simulink model "test07"  (Simulink 7.4)
settings: Solver=ode3  StartTime=0.0  StopTime=inf  RelTol=1e-3
undefined symbols (not defined in the file or in its folder): serial
libraries: instrumentlib x3, NAV420Lib x2, NAV420DecodeLib x1
settings Model: Creator=djulzz  LastModifiedBy=djulzz
settings DebuggingCC: SolverPrmCheckMsg=none

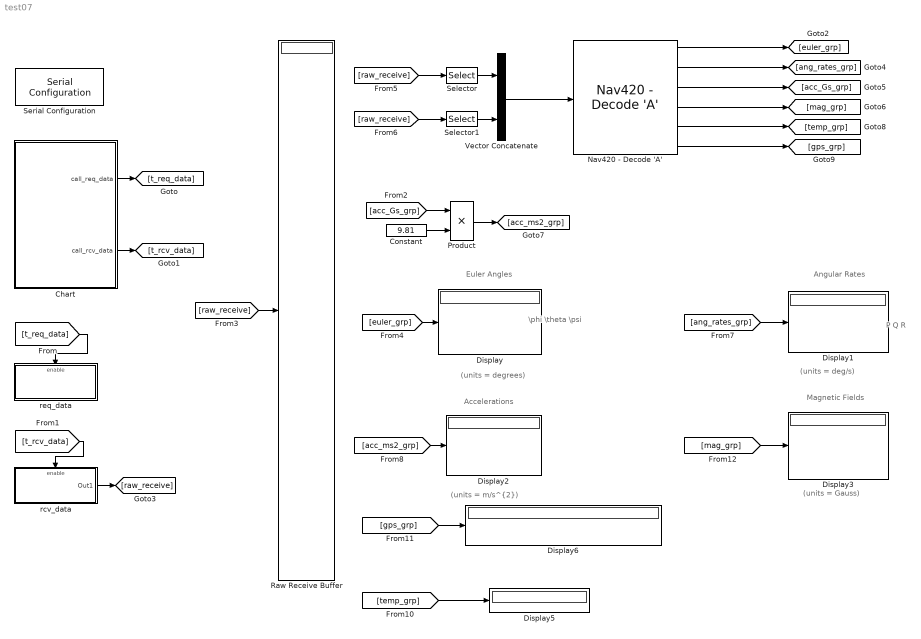
== system test07 ==
  note: \phi
      | \theta
      | \psi
  note: P
      | Q
      | R
  note: (units = degrees)
  note: Euler Angles
  note: Angular Rates
  note: (units = deg/s)
  note: Accelerations
  note: (units = m/s^{2})
  note: (units = Gauss)
  note: Magnetic Fields
  Chart : Stateflow chart
  Constant : Constant  Value=9.81  OutDataTypeMode=double  OutDataType=fixdt(1, 16)  OutScaling=2^0  OutDataTypeStr=double  SampleTime=-1
  Display{,1..3,5..6} (6 alike) : Display
  Nav420 - Decode 'A' : NAV420DecodeLib/Nav420 - Decode 'A'  SystemSampleTime=-1
  Product : Product  OutDataTypeMode=double  OutDataType=fixdt(1, 16)  OutScaling=2^0  OutDataTypeStr=double  RndMeth=Zero
  Raw Receive Buffer : Display
      settings: Format=hex (Stored Integer)  Decimation=35
  Selector : Selector  InputPortWidth=35  IndexOptions=Index vector (dialog)  Indices=[6 7 8 9 10 11 12 13 14 15 16 17 18 19 20 21 22 23 24 25 26 27 28 29 30 31 32 33 34 35]  OutputSizes=1
  Selector1 : Selector  InputPortWidth=35  IndexOptions=Index vector (dialog)  Indices=[1 2 3 4 5]  OutputSizes=1
  Serial Configuration : instrumentlib/Serial Configuration  Priority=-200000  DialogController=instrumentcreatedialog  DialogControllerArgs=DataTag0  ComPortMenu=COM1  ComPort=COM1  ObjConstructor=serial('COM1');  BaudRate=38400  DataBits=8  Parity=none  StopBits=1  FlowControl=none  Timeout=10  ByteOrder=LittleEndian
  Vector Concatenate : Concatenate  Mode=Vector
  rcv_data : Subsystem  TreatAsAtomicUnit=on
  req_data : Subsystem  TreatAsAtomicUnit=on
  wires:
  [t_req_data] -> req_data/Enable
  [t_rcv_data] -> rcv_data/Enable
  Chart/1(call_req_data) -> [t_req_data]
  Chart/2(call_rcv_data) -> [t_rcv_data]
  [raw_receive] -> Raw Receive Buffer/1
  rcv_data/1(Out1) -> [raw_receive]
  Nav420 - Decode 'A'/1 -> [euler_grp]
  [raw_receive] -> Selector/1
  [raw_receive] -> Selector1/1
  Selector1/1 -> Vector Concatenate/2
  Selector/1 -> Vector Concatenate/1
  Vector Concatenate/1 -> Nav420 - Decode 'A'/1
  Nav420 - Decode 'A'/2 -> [ang_rates_grp]
  Nav420 - Decode 'A'/3 -> [acc_Gs_grp]
  Nav420 - Decode 'A'/4 -> [mag_grp]
  Constant/1 -> Product/2
  [acc_Gs_grp] -> Product/1
  Product/1 -> [acc_ms2_grp]
  Nav420 - Decode 'A'/5 -> [temp_grp]
  Nav420 - Decode 'A'/6 -> [gps_grp]
  [euler_grp] -> Display/1
  [ang_rates_grp] -> Display1/1
  [acc_ms2_grp] -> Display2/1
  [gps_grp] -> Display6/1
  [mag_grp] -> Display3/1
  [temp_grp] -> Display5/1

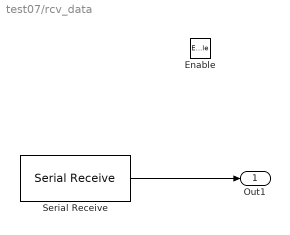
== system test07/rcv_data ==
  Enable : EnablePort
  Serial Receive : instrumentlib/Serial Receive  DialogController=instrumentcreatedialog  DialogControllerArgs=DataTag1  ComPortMenu=COM1  ComPort=COM1  ObjConstructor=serial('COM1');  Terminator=<none>  DataSize="[35   1]"  DataType=uint8  EnableBlockingMode=on  ActionDataUnavailable=Output last received value  CustomValue=0  SampleTime=-1
  Out1 : Outport  DataType=uint8  OutDataType=fixdt(1, 16)  OutScaling=2^0  OutDataTypeStr=uint8
  wires:
  Serial Receive/1 -> Out1/1

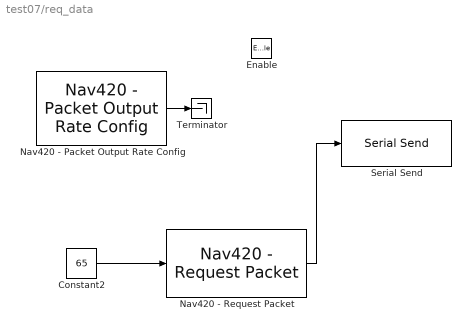
== system test07/req_data ==
  Enable : EnablePort
  Constant2 : Constant  Value=65  OutDataTypeMode=int8  OutDataType=fixdt(1, 16)  OutScaling=2^0  OutDataTypeStr=int8  SampleTime=-1
  Nav420 - Packet Output Rate Config : NAV420Lib/Nav420 - Packet Output Rate Config  SystemSampleTime=-1  shouldSave=on  output_rate=0
  Nav420 - Request Packet : NAV420Lib/Nav420 - Request Packet  SystemSampleTime=-1
  Serial Send : instrumentlib/Serial Send  DialogController=instrumentcreatedialog  DialogControllerArgs=DataTag2  ComPortMenu=COM1  ComPort=COM1  ObjConstructor=serial('COM1');  Terminator=<none>  EnableBlockingMode=on
  Terminator : Terminator
  wires:
  Constant2/1 -> Nav420 - Request Packet/1
  Nav420 - Packet Output Rate Config/1 -> Terminator/1
  Nav420 - Request Packet/1 -> Serial Send/1

== stateflow chart Chart ==
  state Step1
    call_req_data=1;
  state Step2
    call_req_data=0;
  state Step3
    call_rcv_data=1;
  state Step4
    call_rcv_data=0;
  (default) -> Step1
  Step1 -> Step2
  Step2 -> Step3
  Step3 -> Step4
  Step4 -> Step1
  data: call_req_data output uint8; call_rcv_data output uint8
